simulink model "complete_model"  (R2023a)
settings: Solver=VariableStepAuto  StartTime=0.0  StopTime=10.0  RelTol=1e-3
settings Model: Creator=Pedro  LastModifiedBy=Pedro

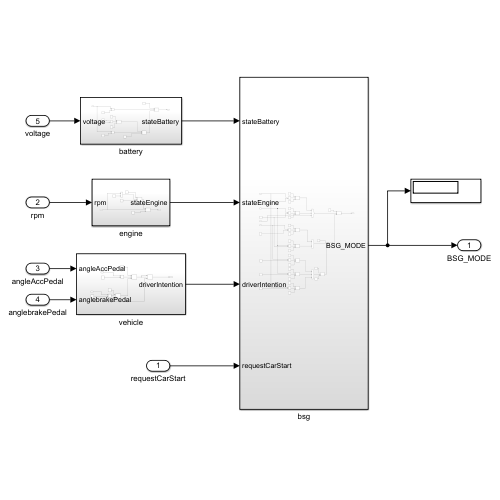
[thumbnail: Simulink's stored preview of the top-level diagram]
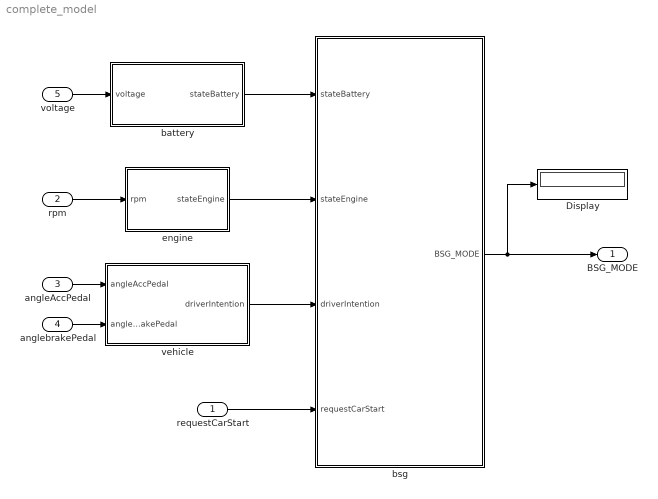
== system complete_model ==
  requestCarStart : Inport
  rpm : Inport  Port=2
  angleAccPedal : Inport  Port=3
  anglebrakePedal : Inport  Port=4
  voltage : Inport  Port=5
  Display : Display
  battery : Subsystem
  bsg : Subsystem
  engine : Subsystem
  vehicle : Subsystem
  BSG_MODE : Outport
  wires:
  bsg/1(BSG_MODE) -> Display/1, BSG_MODE/1
  vehicle/1(driverIntention) -> bsg/3(driverIntention)
  battery/1(stateBattery) -> bsg/1(stateBattery)
  engine/1(stateEngine) -> bsg/2(stateEngine)
  requestCarStart/1 -> bsg/4(requestCarStart)
  rpm/1 -> engine/1(rpm)
  anglebrakePedal/1 -> vehicle/2(anglebrakePedal)
  angleAccPedal/1 -> vehicle/1(angleAccPedal)
  voltage/1 -> battery/1(voltage)

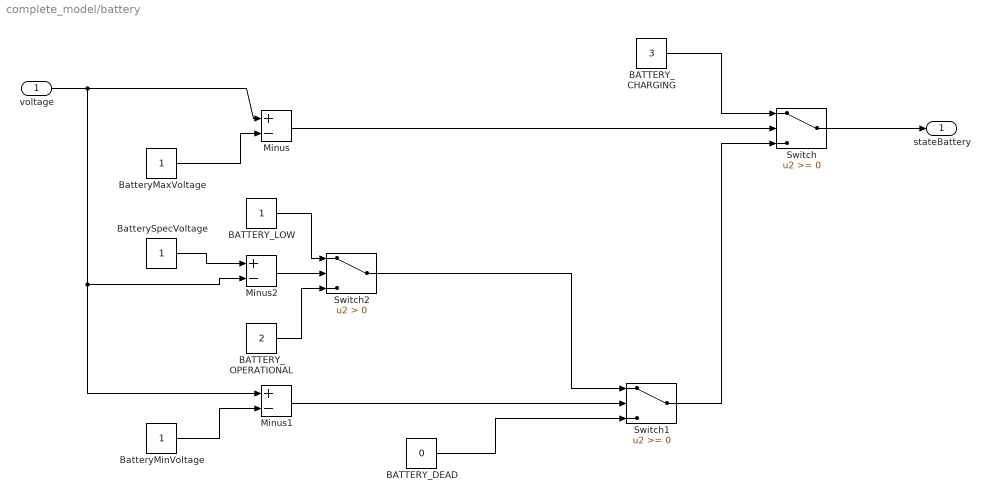
== system complete_model/battery ==
  voltage : Inport
  BATTERY_CHARGING : Constant  Value=3
  BATTERY_DEAD : Constant  Value=0
  BATTERY_LOW : Constant
  BATTERY_OPERATIONAL : Constant  Value=2
  BatteryMaxVoltage : Constant
  BatteryMinVoltage : Constant
  BatterySpecVoltage : Constant
  Minus : Sum  Inputs=+-
  Minus1 : Sum  Inputs=+-
  Minus2 : Sum  Inputs=+-
  Switch : Switch  SaturateOnIntegerOverflow=off  InputSameDT=off
  Switch1 : Switch  SaturateOnIntegerOverflow=off  InputSameDT=off
  Switch2 : Switch  Criteria=u2 > Threshold  SaturateOnIntegerOverflow=off  InputSameDT=off
  stateBattery : Outport
  wires:
  Switch2/1 -> Switch1/1
  BATTERY_OPERATIONAL/1 -> Switch2/3
  BATTERY_CHARGING/1 -> Switch/1
  Minus2/1 -> Switch2/2
  Minus/1 -> Switch/2
  BatteryMaxVoltage/1 -> Minus/2
  voltage/1 -> Minus2/2, Minus1/1, Minus/1
  BatteryMinVoltage/1 -> Minus1/2
  BATTERY_DEAD/1 -> Switch1/3
  Switch1/1 -> Switch/3
  BATTERY_LOW/1 -> Switch2/1
  Minus1/1 -> Switch1/2
  Switch/1 -> stateBattery/1
  BatterySpecVoltage/1 -> Minus2/1

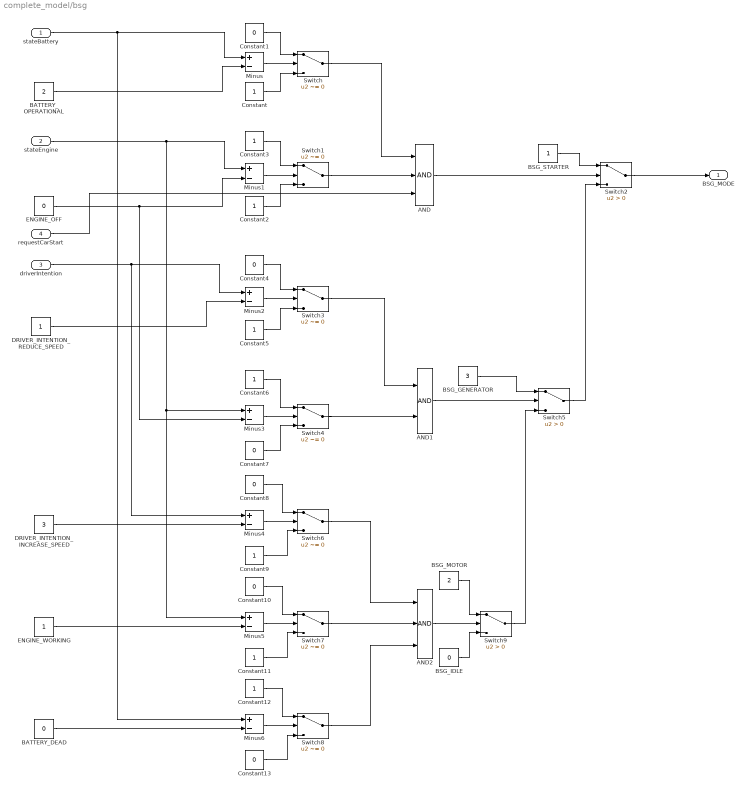
== system complete_model/bsg ==
  stateBattery : Inport
  stateEngine : Inport  Port=2
  driverIntention : Inport  Port=3
  requestCarStart : Inport  Port=4
  AND : Logic  Inputs=3  IconShape=distinctive  AllPortsSameDT=off  OutDataTypeStr=boolean
  AND1 : Logic  IconShape=distinctive  AllPortsSameDT=off  OutDataTypeStr=boolean
  AND2 : Logic  Inputs=3  IconShape=distinctive  AllPortsSameDT=off  OutDataTypeStr=boolean
  BATTERY_DEAD : Constant  Value=0
  BATTERY_OPERATIONAL : Constant  Value=2
  BSG_GENERATOR : Constant  Value=3
  BSG_IDLE : Constant  Value=0
  BSG_MOTOR : Constant  Value=2
  BSG_STARTER : Constant
  Constant{,2..3,5..6,9,11..12} (8 alike) : Constant
  Constant{1,4,7..8,10,13} (6 alike) : Constant  Value=0
  DRIVER_INTENTION_INCREASE_SPEED : Constant  Value=3
  DRIVER_INTENTION_REDUCE_SPEED : Constant
  ENGINE_OFF : Constant  Value=0
  ENGINE_WORKING : Constant  SampleTime=-1
  Minus{,1..6} (7 alike) : Sum  Inputs=+-
  Switch{,1,3..4,6..8} (7 alike) : Switch  Criteria=u2 ~= 0  SaturateOnIntegerOverflow=off  InputSameDT=off
  Switch2 : Switch  Criteria=u2 > Threshold  SaturateOnIntegerOverflow=off  InputSameDT=off
  Switch5 : Switch  Criteria=u2 > Threshold  SaturateOnIntegerOverflow=off  InputSameDT=off
  Switch9 : Switch  Criteria=u2 > Threshold  SaturateOnIntegerOverflow=off  InputSameDT=off
  BSG_MODE : Outport
  wires:
  Constant7/1 -> Switch4/3
  Constant6/1 -> Switch4/1
  stateBattery/1 -> Minus6/1, Minus/1
  Minus5/1 -> Switch7/2
  DRIVER_INTENTION_INCREASE_SPEED/1 -> Minus4/2
  Constant4/1 -> Switch3/1
  BATTERY_OPERATIONAL/1 -> Minus/2
  Switch4/1 -> AND1/2
  stateEngine/1 -> Minus1/1, Minus3/1, Minus5/1
  Minus1/1 -> Switch1/2
  AND/1 -> Switch2/2
  AND1/1 -> Switch5/2
  Minus3/1 -> Switch4/2
  Constant2/1 -> Switch1/3
  BSG_IDLE/1 -> Switch9/3
  ENGINE_OFF/1 -> Minus3/2, Minus1/2
  Constant3/1 -> Switch1/1
  Constant8/1 -> Switch6/1
  Constant9/1 -> Switch6/3
  BATTERY_DEAD/1 -> Minus6/2
  ENGINE_WORKING/1 -> Minus5/2
  Minus/1 -> Switch/2
  Switch8/1 -> AND2/3
  Constant5/1 -> Switch3/3
  Constant10/1 -> Switch7/1
  Switch1/1 -> AND/2
  Minus2/1 -> Switch3/2
  Switch2/1 -> BSG_MODE/1
  Minus6/1 -> Switch8/2
  Constant12/1 -> Switch8/1
  BSG_STARTER/1 -> Switch2/1
  DRIVER_INTENTION_REDUCE_SPEED/1 -> Minus2/2
  Switch6/1 -> AND2/1
  Constant13/1 -> Switch8/3
  Switch7/1 -> AND2/2
  Switch3/1 -> AND1/1
  BSG_GENERATOR/1 -> Switch5/1
  Minus4/1 -> Switch6/2
  AND2/1 -> Switch9/2
  Switch5/1 -> Switch2/3
  driverIntention/1 -> Minus4/1, Minus2/1
  Constant11/1 -> Switch7/3
  Switch/1 -> AND/1
  Switch9/1 -> Switch5/3
  requestCarStart/1 -> AND/3
  Constant/1 -> Switch/3
  BSG_MOTOR/1 -> Switch9/1
  Constant1/1 -> Switch/1

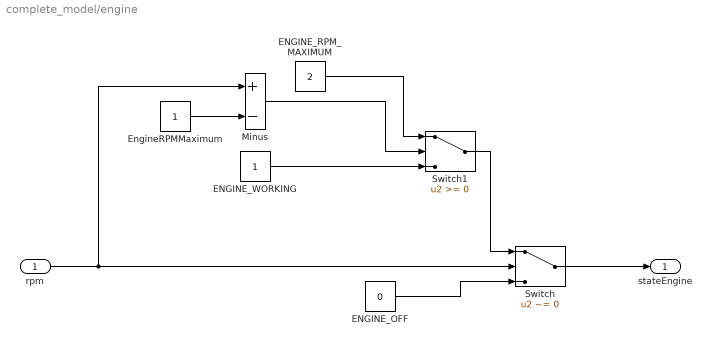
== system complete_model/engine ==
  rpm : Inport
  ENGINE_OFF : Constant  Value=0
  ENGINE_RPM_MAXIMUM : Constant  Value=2
  ENGINE_WORKING : Constant
  EngineRPMMaximum : Constant
  Minus : Sum  Inputs=+-
  Switch : Switch  Criteria=u2 ~= 0  SaturateOnIntegerOverflow=off  InputSameDT=off
  Switch1 : Switch  SaturateOnIntegerOverflow=off  InputSameDT=off
  stateEngine : Outport
  wires:
  Switch1/1 -> Switch/1
  rpm/1 -> Switch/2, Minus/1
  ENGINE_RPM_MAXIMUM/1 -> Switch1/1
  ENGINE_WORKING/1 -> Switch1/3
  EngineRPMMaximum/1 -> Minus/2
  ENGINE_OFF/1 -> Switch/3
  Switch/1 -> stateEngine/1
  Minus/1 -> Switch1/2

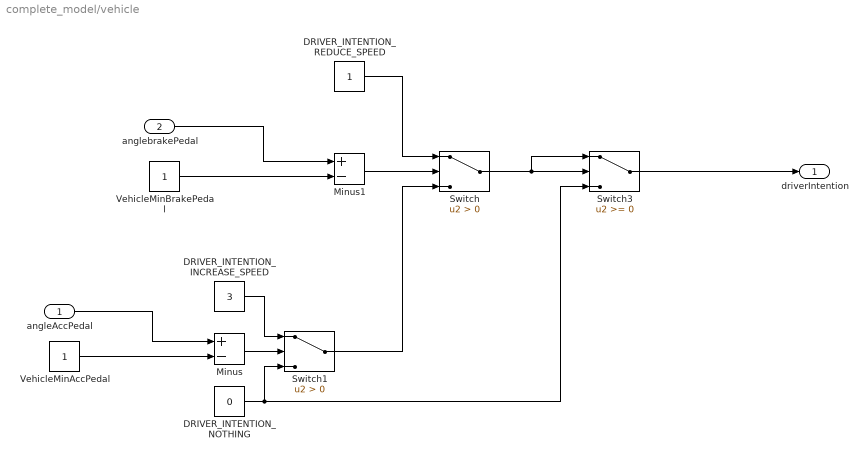
== system complete_model/vehicle ==
  angleAccPedal : Inport
  anglebrakePedal : Inport  Port=2
  DRIVER_INTENTION_INCREASE_SPEED : Constant  Value=3
  DRIVER_INTENTION_NOTHING : Constant  Value=0
  DRIVER_INTENTION_REDUCE_SPEED : Constant
  Minus : Sum  Inputs=+-
  Minus1 : Sum  Inputs=+-
  Switch : Switch  Criteria=u2 > Threshold  SaturateOnIntegerOverflow=off  InputSameDT=off
  Switch1 : Switch  Criteria=u2 > Threshold  SaturateOnIntegerOverflow=off  InputSameDT=off
  Switch3 : Switch  SaturateOnIntegerOverflow=off  InputSameDT=off
  VehicleMinAccPedal : Constant
  VehicleMinBrakePedal : Constant
  driverIntention : Outport
  wires:
  DRIVER_INTENTION_NOTHING/1 -> Switch1/3, Switch3/3
  Switch3/1 -> driverIntention/1
  Switch/1 -> Switch3/1, Switch3/2
  Switch1/1 -> Switch/3
  DRIVER_INTENTION_INCREASE_SPEED/1 -> Switch1/1
  VehicleMinBrakePedal/1 -> Minus1/2
  VehicleMinAccPedal/1 -> Minus/2
  Minus/1 -> Switch1/2
  anglebrakePedal/1 -> Minus1/1
  angleAccPedal/1 -> Minus/1
  Minus1/1 -> Switch/2
  DRIVER_INTENTION_REDUCE_SPEED/1 -> Switch/1
